simulink model "kelvinVoigtTether_th2"  (R2018b)
settings: Solver=VariableStepAuto  StartTime=0.0  StopTime=10  RelTol=1e-3
undefined symbols (not defined in the file or in its folder): class_thr
libraries: kelvinVoigtTether_cl x1
settings Model: Creator=Ayaz  LastModifiedBy=Ayaz

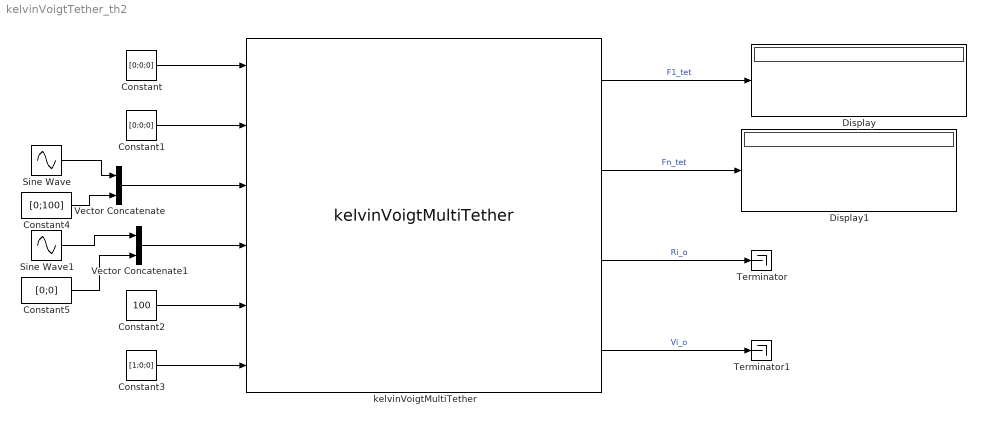
== system kelvinVoigtTether_th2 ==
  Constant : Constant  Value=[0;0;0]  VectorParams1D=off
  Constant1 : Constant  Value=[0;0;0]  VectorParams1D=off
  Constant2 : Constant  Value=100
  Constant3 : Constant  Value=[1;0;0]  VectorParams1D=off
  Constant4 : Constant  Value=[0;100]  VectorParams1D=off
  Constant5 : Constant  Value=[0;0]  VectorParams1D=off
  Display : Display
  Display1 : Display
  Sine Wave : Sin  Amplitude=5  SampleTime=0
  Sine Wave1 : Sin  Amplitude=5  Phase=pi/2  SampleTime=0
  Terminator : Terminator
  Terminator1 : Terminator
  Vector Concatenate : Concatenate
  Vector Concatenate1 : Concatenate
  kelvinVoigtMultiTether : kelvinVoigtTether_cl/kelvinVoigtMultiTether  rho_fluid=rho_f  grav=G  M=mass  tN=[class_thr.numNodes]  tD=[class_thr.diameter]  tRho=[class_thr.density]  tE=[class_thr.youngsModulus]  tZeta=[class_thr.dampingRatio]  tCd=[class_thr.dragCoeff]  iniR1_o=[class_thr.ini_R1_o]  iniRn_o=[class_thr.ini_Rn_o]  iniRi_o=n_ini_pos  iniVi_o=n_ini_vel
  wires:
  kelvinVoigtMultiTether/3 -> Terminator/1  "Ri_o"
  kelvinVoigtMultiTether/1 -> Display/1  "F1_tet"
  kelvinVoigtMultiTether/2 -> Display1/1  "Fn_tet"
  kelvinVoigtMultiTether/4 -> Terminator1/1  "Vi_o"
  Constant/1 -> kelvinVoigtMultiTether/1
  Constant1/1 -> kelvinVoigtMultiTether/2
  Constant2/1 -> kelvinVoigtMultiTether/5
  Constant3/1 -> kelvinVoigtMultiTether/6
  Vector Concatenate/1 -> kelvinVoigtMultiTether/3
  Sine Wave/1 -> Vector Concatenate/1
  Constant4/1 -> Vector Concatenate/2
  Constant5/1 -> Vector Concatenate1/2
  Sine Wave1/1 -> Vector Concatenate1/1
  Vector Concatenate1/1 -> kelvinVoigtMultiTether/4
